simulink model "vx_vy_lifesig_fusion_v2_8a2_long_low_yaw"  (R2024a)
settings: Solver=VariableStepAuto  StartTime=0.0  StopTime=22  RelTol=1e-3
model workspace (MAT data in the model file):
  ax_imu_prereq_Ts = 0.01
  ax_imu_prereq_bias = 0.02
  ax_imu_prereq_fc = 20
  ax_imu_prereq_noise_variance = 2.5e-05
  long_low_yaw_excitation_end_s = 4.5
  long_low_yaw_initial_straight_s = 2
  long_low_yaw_sample_time = 0.01
  long_low_yaw_steer_amplitude_rad = 0.02
  long_low_yaw_steer_frequency_hz = 0.4
  long_low_yaw_steer_profile = [0 0.01 0.02 0.03 0.04 0.05 0.06 0.07 0.08 0.09 0.1 0.11 ... (4402 elements, 2201x2)]
  long_low_yaw_stop_time = 22
  test_steer_amplitude = 0.02
  test_steer_frequency = 0.4
  vy_v17_mode_code = 20
undefined symbols (not defined in the file or in its folder): longitudinal_velocity_estimator_simulink, vy_dynamic_ekf, vy_dynamic_ekf_v1_17_reliability_numeric
libraries: simulink x6, Solver_SF x1
(part 1 of 2)
Description:
  | V2.5 FIXED-WEIGHT INTEGRATION TARGET. Fusion weights [1/3 1/3 1/3] are TEST-ONLY, NOT SELECTED BASELINE WEIGHTS, NOT TUNED, and NOT FROZEN. F P0_F=0.5 and Q_F=0.0025 remain TEST-ONLY, UNTUNED, and UNFROZEN. F feedback_valid_current is fixed false; Vy_FW is observation-only and is not fed back. V2.7 reliability capture role: NON_HOLDOUT_ENGINEERING_DIAGNOSTIC. It is not H01/H02/H03 and must not overwrite formal holdout evidence.
  | V2.7 LIFESIG INTEGRATION TARGET. Independent observation-only LifeSig fusion. Formal fusion inputs are Vy_D/update_valid_D, Vy_K/update_valid_K, Vy_F/propagation_age_steps/age_valid_F, and reset only. NIS, yaw observability, disagreement, covariance, and online truth are excluded. Existing F runtime parameters remain P0_F=0.5 and Q_F=0.0025.
  | V2.8-A2 NON-HOLDOUT LONG-LOW-YAW VALIDATION TARGET. 100-Hz steering: 2.0 s exact zero, one 0.02-rad 0.4-Hz sine period, then 17.5 s exact zero. Vy_true and D/K errors are observation-only diagnostics. No K gate is implemented.
settings Model: Creator=Xiao Hu  LastModifiedBy=21180

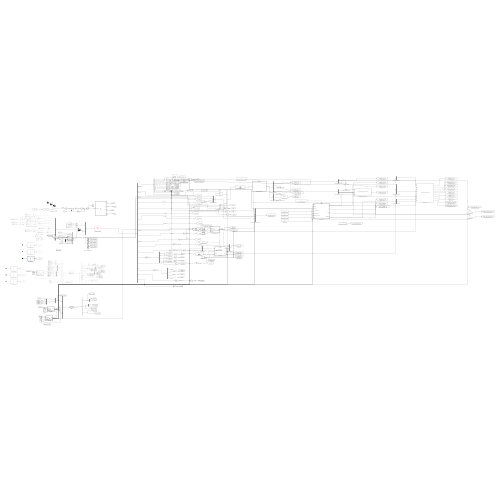
[thumbnail: Simulink's stored preview of the top-level diagram]
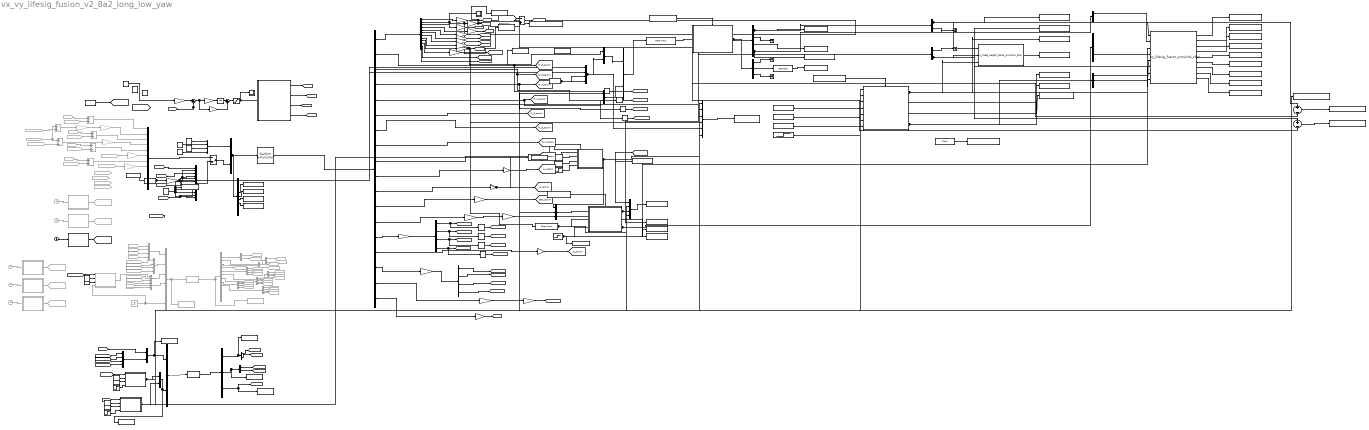
== system vx_vy_lifesig_fusion_v2_8a2_long_low_yaw ==
  note: Product
  AVz传感器 : MATLAB Function  TreatAsAtomicUnit=on  SystemSampleTime=0.01
  Add1 : Sum  Inputs=-+
  Add{4..9} (6 alike) : Sum  Commented=on
  Ax Clean 100Hz Log : ToWorkspace  VariableName=ax_clean_100hz_prereq_log1  SaveFormat=Timeseries  SampleTime=-1
  Ax IMU Bias : Constant  Value=0.02
  Ax IMU Input RT 100Hz : RateTransition  OutPortSampleTime=0.01
  Ax IMU Log : ToWorkspace  VariableName=ax_imu_prereq_log1  SaveFormat=Timeseries  SampleTime=-1
  Ax IMU Reset : Step  Time=0.01  Before=1  After=0  SampleTime=0
  Ax IMU Sensor 100Hz : MATLAB Function  TreatAsAtomicUnit=on  SystemSampleTime=0.01
  Ax IMU White Noise : RandomNumber  Variance=0.000025  Seed=20260820  SampleTime=0.01
  B高附着加速 : MATLAB Function  Commented=on  TreatAsAtomicUnit=on
  CarSim S-Function : Solver_SF/CarSim S-Function  Priority=1  SIMFILE=simfile.sim  Run_RTs=off  vs_state_ind=Run  StopMode_ind=Vehicle Model
  Clock{,1,3..5} (5 alike) : Clock  Commented=on
  Clock2 : Clock
  Constant : Constant  Value=0.02
  Constant1 : Constant  Value=0.02
  Constant{6..10} (5 alike) : Constant  Value=0
  Constant2 : Constant  Value=0.005
  Constant4 : Constant  Value=0.8
  C高附着减速 : MATLAB Function  Commented=on  TreatAsAtomicUnit=on
  D LifeSig Valid Demux : Demux  Outputs=[1 1]
  Demux : Demux  Commented=on  Outputs=[2 2 2 1 4 4 4 4 4 2 2 7]
  Demux{1,9..11,13} (5 alike) : Demux  Commented=on
  Demux12 : Demux  Outputs=[2 2 9]
  Demux14 : Demux  Outputs=2
  Demux18 : Demux  Outputs=2
  Demux2 : Demux  Commented=on  Outputs=2
  Demux3 : Demux
  Demux4 : Demux  Outputs=12
  Demux5 : Demux  Outputs=[12 1 1 1 1 1 1 1 1 1 1 1 1 4 1 4 1 1]
  Demux6 : Demux
  Demux7 : Demux  Commented=on  Outputs=2
  Demux8 : Demux  Commented=on  Outputs=2
  Derivative{,1..4,6..7,12} (8 alike) : Derivative
  D高附着加减速1 : MATLAB Function  TreatAsAtomicUnit=on
  F Feedback Valid Disabled : Constant  Value=0  OutDataTypeStr=double  SampleTime=0.01
  F LifeSig Reliability Demux : Demux  Outputs=[1 1 1]
  F P Feedback Placeholder : Constant  Value=0.5  OutDataTypeStr=double  SampleTime=0.01
  F Reset First Hit : Step  Time=0.01  Before=1  After=0  SampleTime=0.01
  F Vy Feedback Placeholder : Constant  Value=0  OutDataTypeStr=double  SampleTime=0.01
  F-Track 100Hz : Subsystem  TreatAsAtomicUnit=on
  F-Track 100Hz Scheduler : simulink/Ports & Subsystems/Function-Call Generator  sample_time=0.01  numberOfIterations=1  DisallowWideOutput=off
  Fixed Weight D K F Fusion : M-S-Function  FunctionName=vy_fixed_weight_fusion_simulink_sfun  Parameters=0.9004680917645591,1-0.9004680917645591,0
  From : From  Commented=on  GotoTag=weelrate_fl  TagVisibility=global
  From11 : From  Commented=on  GotoTag=weelrate_fr  TagVisibility=global
  From12 : From  Commented=on  GotoTag=W5_T  TagVisibility=global
  From13 : From  Commented=on  GotoTag=W1_T  TagVisibility=global
  From14 : From  Commented=on  GotoTag=weelrate_rl  TagVisibility=global
  From15 : From  Commented=on  GotoTag=weelrate_rr  TagVisibility=global
  From16 : From  Commented=on  GotoTag=WEEL1  TagVisibility=global
  From17 : From  Commented=on  GotoTag=WEEL3  TagVisibility=global
  From18 : From  Commented=on  GotoTag=WEEL2  TagVisibility=global
  From19 : From  Commented=on  GotoTag=WEEL4  TagVisibility=global
  From2 : From  Commented=on  GotoTag=Fd2  TagVisibility=global
  From20 : From  Commented=on  GotoTag=yawrate  TagVisibility=global
  From21 : From  Commented=on  GotoTag=W3_T  TagVisibility=global
  From22 : From  Commented=on  GotoTag=Delta_Torque_rl  TagVisibility=global
  From23 : From  Commented=on  GotoTag=Delta_Torque_fr  TagVisibility=global
  From24 : From  Commented=on  GotoTag=Delta_Torque_rr  TagVisibility=global
  From25 : From  Commented=on  GotoTag=rollrate  TagVisibility=global
  From26 : From  Commented=on  GotoTag=Ay_carsim  TagVisibility=global
  From28 : From  Commented=on  GotoTag=Az_carsim  TagVisibility=global
  From29 : From  Commented=on  GotoTag=W7_T  TagVisibility=global
  From3 : From  Commented=on  GotoTag=Delta_Torque_fl  TagVisibility=global
  From30 : From  Commented=on  GotoTag=pitchrate  TagVisibility=global
  From35 : From  Commented=on  GotoTag=driver_steering
  From39 : From  Commented=on  GotoTag=Delta_Steering_rl  TagVisibility=global
  From4 : From  Commented=on  GotoTag=Fd3  TagVisibility=global
  From42 : From  Commented=on  GotoTag=Delta_Steering_rr  TagVisibility=global
  From43 : From  Commented=on  GotoTag=Fd1  TagVisibility=global
  From5 : From  Commented=on  GotoTag=Delta_Steering_fl  TagVisibility=global
  From50 : From  Commented=on  GotoTag=Fd4  TagVisibility=global
  From6 : From  Commented=on  GotoTag=Delta_Steering_fr  TagVisibility=global
  Fusion D State Select Vy : Demux  Outputs=2
  Fusion D r Terminator : Terminator
  Fusion K State Select Vy : Demux  Outputs=2
  Fusion K Vx Terminator : Terminator
  F低附着加速1 : MATLAB Function  Commented=on  TreatAsAtomicUnit=on
  F低附着加速2 : MATLAB Function  Commented=on  TreatAsAtomicUnit=on
  G0 CarSim Input Demux : Demux  Outputs=16
  G0 Steer Cmd Rad : FromWorkspace  VariableName=long_low_yaw_steer_profile  SampleTime=0.01  Interpolate=off  OutputAfterFinalValue=Holding final value
  Gain{1,10,12,14,17..18,23,29,37} (9 alike) : Gain  Gain=pi/180
  Gain11 : Gain  Gain=1/3.6
  Gain{3,5,9,13} (4 alike) : Gain  Commented=on  Gain=180/pi
  Gain15 : Gain  Gain=1/3.6
  Gain16 : Gain  Gain=9.8
  Gain19 : Gain  Gain=1/16.8
  Gain2 : Gain  Gain=1/16.8
  Gain21 : Gain  Gain=5000
  Gain22 : Gain  Gain=180/pi
  Gain{6..8,24} (4 alike) : Gain  Gain=pi/30
  Gain25 : Gain  Gain=0.07
  Gain28 : Gain  Gain=9.8
  Gain36 : Gain  Gain=9.8
  Gain38 : Gain  Gain=1/3.6
  Gain39 : Gain  Commented=on
  Gain4 : Gain  Gain=1/1000
  Goto10 : Goto  Commented=on  GotoTag=vx_wss  TagVisibility=global
  Goto17 : Goto  Commented=on  GotoTag=P_wss  TagVisibility=global
  Goto28 : Goto  Commented=on  GotoTag=vx_imu  TagVisibility=global
  Goto29 : Goto  Commented=on  GotoTag=P_imu  TagVisibility=global
  Goto30 : Goto  Commented=on  GotoTag=P_wss_imu  TagVisibility=global
  Goto32 : Goto  Commented=on  GotoTag=vx_FL  TagVisibility=global
  Goto38 : Goto  Commented=on  GotoTag=vx_FR  TagVisibility=global
  Goto39 : Goto  Commented=on  GotoTag=vx_RL  TagVisibility=global
  Goto40 : Goto  Commented=on  GotoTag=vx_RR  TagVisibility=global
  Goto41 : Goto  Commented=on  GotoTag=slip_FL  TagVisibility=global
  Goto57 : Goto  Commented=on  GotoTag=slip_FR  TagVisibility=global
  Goto58 : Goto  Commented=on  GotoTag=slip_RL  TagVisibility=global
  Goto59 : Goto  Commented=on  GotoTag=slip_RR  TagVisibility=global
  Goto64 : Goto  Commented=on  GotoTag=rho_FL  TagVisibility=global
  Goto65 : Goto  Commented=on  GotoTag=rho_FR  TagVisibility=global
  Goto66 : Goto  Commented=on  GotoTag=rho_RL  TagVisibility=global
  Goto67 : Goto  Commented=on  GotoTag=rho_RR  TagVisibility=global
  Goto68 : Goto  Commented=on  GotoTag=R_FL  TagVisibility=global
  Goto69 : Goto  Commented=on  GotoTag=R_FR  TagVisibility=global
  Goto7 : Goto  Commented=on  GotoTag=vx_hat  TagVisibility=global
  Goto70 : Goto  Commented=on  GotoTag=R_RL  TagVisibility=global
  Goto71 : Goto  Commented=on  GotoTag=R_RR  TagVisibility=global
  Goto72 : Goto  Commented=on  GotoTag=R_FL  TagVisibility=global
  Goto73 : Goto  Commented=on  GotoTag=R_FR  TagVisibility=global
  Goto74 : Goto  Commented=on  GotoTag=R_RL  TagVisibility=global
  Goto75 : Goto  Commented=on  GotoTag=R_RR  TagVisibility=global
  Goto{76..77,80..82} (5 alike) : Goto  Commented=on  GotoTag=vx_ref  TagVisibility=global
  Goto9 : Goto  Commented=on  GotoTag=P_fused  TagVisibility=global
  G低附着减速2 : MATLAB Function  Commented=on  TreatAsAtomicUnit=on
  H低附着加减速 : MATLAB Function  Commented=on  TreatAsAtomicUnit=on
  Integrator1 : Integrator
  K LifeSig Diagnostic Demux : Demux  Outputs=[1 1 1 1 1 1 1]
  K-KF 100Hz : Subsystem  TreatAsAtomicUnit=on
  K-KF 100Hz Scheduler : simulink/Ports & Subsystems/Function-Call Generator  sample_time=0.01  numberOfIterations=1  DisallowWideOutput=off
  K-KF IMU Mux : Mux  Inputs=3
  K-KF Input Log Mux : Mux
  K-KF P Log : ToWorkspace  VariableName=kkf_P_log1  SaveFormat=Timeseries  SampleTime=-1
  K-KF Reset First Call : Step  Time=0.01  Before=1  After=0  SampleTime=0.01
  K-KF Vx RT 100Hz : RateTransition  OutPortSampleTime=0.01
  K-KF diag Log : ToWorkspace  VariableName=kkf_diag_log1  SaveFormat=Timeseries  SampleTime=-1
  K-KF u Log : ToWorkspace  VariableName=kkf_u_log1  SaveFormat=Timeseries  SampleTime=-1
  K-KF x Log : ToWorkspace  VariableName=kkf_x_log1  SaveFormat=Timeseries  SampleTime=-1
  LifeSig D K F Fusion : M-S-Function  FunctionName=vy_lifesig_fusion_simulink_sfun
  Long Low Yaw D Error : Sum  Inputs=+-
  Long Low Yaw D Error Log : ToWorkspace  VariableName=long_low_yaw_d_error_log  SaveFormat=Timeseries  SampleTime=-1
  Long Low Yaw K Error : Sum  Inputs=+-
  Long Low Yaw K Error Log : ToWorkspace  VariableName=long_low_yaw_k_error_log  SaveFormat=Timeseries  SampleTime=-1
  Long Low Yaw Signed r Log : ToWorkspace  VariableName=long_low_yaw_r_log  SaveFormat=Timeseries  SampleTime=-1
  MATLAB Function5 : MATLAB Function  TreatAsAtomicUnit=on
  Manual Switch1 : ManualSwitch  CurrentSetting=0
  Mux : Mux  Commented=on  Inputs=[4 4 3 3 3 1]
  Mux1 : Mux  Commented=on
  Mux10 : Mux  Inputs=[1 4]
  Mux11 : Mux
  Mux12 : Mux  Inputs=2
  Mux2 : Mux  Commented=on
  Mux3 : Mux  Commented=on  Inputs=3
  Mux4 : Mux  Commented=on  Inputs=3
  Mux5 : Mux  Inputs=12
  Mux6 : Mux
  Mux7 : Mux  Inputs=[4,12]
  Mux8 : Mux  Inputs=12
  Mux9 : Mux  Inputs=[5 2]
  Parallel D Control Mux : Mux  Inputs=[1 4]
  Parallel D Full P Extract : Demux  Outputs=[45 4 22]
  Parallel D Input Mux : Mux  Inputs=[5 2]
  Parallel D Measurement Mux : Mux  Inputs=2
  Parallel D Output Demux : Demux  Outputs=[2 2 65 2]
  Parallel D P 2x2 : Reshape  OutputDimensionality=Customize  OutputDimensions=[2 2]
  Parallel D P Head Terminator : Terminator
  Parallel D P Tail Terminator : Terminator
  Parallel D Pdiag Terminator : Terminator
  Parallel D Rear Steer Zero Rad : Constant  Value=0  OutDataTypeStr=double
  Parallel D Steering Mux : Mux
  Parallel D-EKF 100Hz : Subsystem  TreatAsAtomicUnit=on
  Parallel D-EKF 100Hz Scheduler : simulink/Ports & Subsystems/Function-Call Generator  sample_time=0.01  numberOfIterations=1  DisallowWideOutput=off
  Parallel D-EKF Input RT 100Hz : RateTransition  OutPortSampleTime=0.01
  Parallel Physical Input Log Mux : Mux  Inputs=[1 1 1 1 4 1]
  Random Number : RandomNumber  Variance=0.000025  Seed=20260819  SampleTime=0.01
  Random Number1 : RandomNumber  Variance=0.000025  Seed=20260819  SampleTime=0.01
  Random Number2 : RandomNumber  Variance=0.000025  Seed=20260819  SampleTime=0.01
  Reliability Common Time 100Hz : DigitalClock  SampleTime=0.01
  Reliability Common Time Log : ToWorkspace  VariableName=rel_common_time_100hz_log  SaveFormat=Timeseries  SampleTime=-1
  Reliability D Valid Log : ToWorkspace  VariableName=rel_d_valid_log  SaveFormat=Timeseries  SampleTime=-1
  Reliability F Diagnostic Log : ToWorkspace  VariableName=rel_f_reliability_log  SaveFormat=Timeseries  SampleTime=-1
  Reliability Vy True 100Hz Log : ToWorkspace  VariableName=rel_vy_true_100hz_log  SaveFormat=Timeseries  SampleTime=-1
  Reliability Vy True RT 100Hz : RateTransition  OutPortSampleTime=0.01
  Repeating Sequence Interpolated : simulink/Sources/Repeating Sequence Interpolated  OutValues=[40 40 40 40].'  TimeValues=[0 3 8 16].'  LookUpMeth=Interpolation-Use End Values  tsamp=0.001  OutMin=[]  OutMax=[]  OutDataTypeStr=double  OutputDataTypeScalingMode=double  OutDataType=fixdt(0,8)  OutScaling=2^-10
  Repeating Sequence Interpolated1 : simulink/Sources/Repeating Sequence Interpolated  OutValues=[60 60 60 60].'  TimeValues=[0 3 8 16].'  LookUpMeth=Interpolation-Use End Values  tsamp=0.001  OutMin=[]  OutMax=[]  OutDataTypeStr=double  OutputDataTypeScalingMode=double  OutDataType=fixdt(0,8)  OutScaling=2^-10
  Repeating Sequence Interpolated2 : simulink/Sources/Repeating Sequence Interpolated  OutValues=[72 72 72 72].'  TimeValues=[0 3 8 16].'  LookUpMeth=Interpolation-Use End Values  tsamp=0.001  OutMin=[]  OutMax=[]  OutDataTypeStr=double  OutputDataTypeScalingMode=double  OutDataType=fixdt(0,8)  OutScaling=2^-10
  Saturation : Saturate  UpperLimit=2250  LowerLimit=-2250
  Scope3 : Scope
  Scope8 : Scope
  Step : Step  Commented=on  Time=0.01  Before=1  After=0  SampleTime=0
  Step1 : Step  Time=0.01  Before=1  After=0  SampleTime=0
  Step2 : Step  Time=0.01  Before=1  After=0  SampleTime=0
  Sum3 : Sum  Inputs=|+-
  Sum4 : Sum  Inputs=|++
  To Workspace : ToWorkspace  Commented=on  VariableName=est_y_log  SaveFormat=Timeseries  SampleTime=-1
  To Workspace1 : ToWorkspace  Commented=on  VariableName=est_u_log  SaveFormat=Timeseries  SampleTime=-1
  To Workspace10 : ToWorkspace  VariableName=avz_log1  SaveFormat=Timeseries  SampleTime=-1
  To Workspace2 : ToWorkspace  VariableName=Vx_true_log  SaveFormat=Timeseries  SampleTime=-1
  To Workspace3 : ToWorkspace  VariableName=est_y_log1  SaveFormat=Timeseries  SampleTime=-1
  To Workspace4 : ToWorkspace  VariableName=est_u_log1  SaveFormat=Timeseries  SampleTime=-1
  To Workspace5 : ToWorkspace  VariableName=Vx_true_log2  SaveFormat=Timeseries  SampleTime=-1
  To Workspace6 : ToWorkspace  VariableName=est_z_log1  SaveFormat=Timeseries  SampleTime=-1
  To Workspace7 : ToWorkspace  VariableName=est_diag_log1  SaveFormat=Timeseries  SampleTime=-1
  To Workspace8 : ToWorkspace  VariableName=est_P_log1  SaveFormat=Timeseries  SampleTime=-1
  To Workspace9 : ToWorkspace  VariableName=vy_true_log1  SaveFormat=Timeseries  SampleTime=-1
  avz_imu_g0 : ToWorkspace  VariableName=avz_imu_g0  SaveFormat=Timeseries  SampleTime=-1
      settings: MaxDataPoints=100000
  ay传感器 : MATLAB Function  TreatAsAtomicUnit=on  SystemSampleTime=0.01
  dekf_P_log : ToWorkspace  VariableName=dekf_P_log  SaveFormat=Timeseries  SampleTime=-1
      settings: MaxDataPoints=100000
  dekf_diag_log : ToWorkspace  VariableName=dekf_diag_log  SaveFormat=Timeseries  SampleTime=-1
      settings: MaxDataPoints=100000
  dekf_x_log : ToWorkspace  VariableName=dekf_x_log  SaveFormat=Timeseries  SampleTime=-1
      settings: MaxDataPoints=100000
  fusion_f_P_log : ToWorkspace  VariableName=fusion_f_P_log  SaveFormat=Timeseries  SampleTime=-1
  fusion_f_diag_log : ToWorkspace  VariableName=fusion_f_diag_log  SaveFormat=Timeseries  SampleTime=-1
  fusion_vy_d_log : ToWorkspace  VariableName=fusion_vy_d_log  SaveFormat=Timeseries  SampleTime=-1
  fusion_vy_f_log : ToWorkspace  VariableName=fusion_vy_f_log  SaveFormat=Timeseries  SampleTime=-1
  fusion_vy_fw_log : ToWorkspace  VariableName=fusion_vy_fw_log  SaveFormat=Timeseries  SampleTime=-1
  fusion_vy_k_log : ToWorkspace  VariableName=fusion_vy_k_log  SaveFormat=Timeseries  SampleTime=-1
  lifesig_alpha_d_log : ToWorkspace  VariableName=lifesig_alpha_d_log  SaveFormat=Timeseries  SampleTime=-1
  lifesig_alpha_f_log : ToWorkspace  VariableName=lifesig_alpha_f_log  SaveFormat=Timeseries  SampleTime=-1
  lifesig_alpha_k_log : ToWorkspace  VariableName=lifesig_alpha_k_log  SaveFormat=Timeseries  SampleTime=-1
  lifesig_fallback_active_log : ToWorkspace  VariableName=lifesig_fallback_active_log  SaveFormat=Timeseries  SampleTime=-1
  lifesig_fusion_valid_log : ToWorkspace  VariableName=lifesig_fusion_valid_log  SaveFormat=Timeseries  SampleTime=-1
  lifesig_h_d_log : ToWorkspace  VariableName=lifesig_h_d_log  SaveFormat=Timeseries  SampleTime=-1
  lifesig_h_f_log : ToWorkspace  VariableName=lifesig_h_f_log  SaveFormat=Timeseries  SampleTime=-1
  lifesig_h_k_log : ToWorkspace  VariableName=lifesig_h_k_log  SaveFormat=Timeseries  SampleTime=-1
  lifesig_vy_ls_log : ToWorkspace  VariableName=lifesig_vy_ls_log  SaveFormat=Timeseries  SampleTime=-1
  parallel_input_log : ToWorkspace  VariableName=parallel_input_log  SaveFormat=Timeseries  SampleTime=-1
      settings: MaxDataPoints=100000
  reset_g0 : ToWorkspace  VariableName=reset_g0  SaveFormat=Timeseries  SampleTime=-1
      settings: MaxDataPoints=100000
  steer_cmd_rad : ToWorkspace  VariableName=steer_cmd_rad  SaveFormat=Timeseries  SampleTime=-1
      settings: MaxDataPoints=100000
  steer_fl_carsim_deg : ToWorkspace  VariableName=steer_fl_carsim_deg  SaveFormat=Timeseries  SampleTime=-1
      settings: MaxDataPoints=100000
  steer_fr_carsim_deg : ToWorkspace  VariableName=steer_fr_carsim_deg  SaveFormat=Timeseries  SampleTime=-1
      settings: MaxDataPoints=100000
  steer_rl_carsim_deg : ToWorkspace  VariableName=steer_rl_carsim_deg  SaveFormat=Timeseries  SampleTime=-1
      settings: MaxDataPoints=100000
  steer_rr_carsim_deg : ToWorkspace  VariableName=steer_rr_carsim_deg  SaveFormat=Timeseries  SampleTime=-1
      settings: MaxDataPoints=100000
  steer_to_carsim_deg : ToWorkspace  VariableName=steer_to_carsim_deg  SaveFormat=Timeseries  SampleTime=-1
      settings: MaxDataPoints=100000
  估计vx : MATLABFcn  Commented=on  MATLABFcn=longitudinal_velocity_estimator_simulink(u)  OutputDimensions=38
  估计vy : MATLABFcn  MATLABFcn=vy_dynamic_ekf(u)  OutputDimensions=13
  tag scope: Ax_carsim=global, Ay_carsim=global, Az_carsim=global, Fx_fl_carsim=global, Fx_fr_carsim=global, Fx_rl_carsim=global, Fx_rr_carsim=global, Fy_fl_carsim=global, Fy_fr_carsim=global, Fy_rl_carsim=global, Fy_rr_carsim=global, P_r=global, P_vy=global, Vx=global, Vy=global, Vy_hat=global, W1_T=global, W3_T=global, W5_T=global, W7_T=global, WEEL1=global, WEEL2=global, WEEL3=global, WEEL4=global, beta_carsim=global, delta_zs1=global, delta_zs2=global, delta_zs3=global, delta_zs4=global, delta_zsd1=global, delta_zsd2=global, delta_zsd3=global, delta_zsd4=global, diag_out=global, driver_steering10=global, driver_steering5=global, e_yawrate=global, fyd1=global, fyd2=global, fyd3=global, fyd4=global, mu=global, pitchrate=global, r_hat=global, roll=global, rollrate=global, vx_ref=global, weelrate_fl=global, weelrate_fr=global, weelrate_rl=global, weelrate_rr=global, x_carsim=global, y_carsim=global, yaw_carsim=global, yawrate=global
  wires:
  From13/1 -> Add4/1
  Gain14/1 -> Gain2/1  "beta_carsim"
  Add1/1 -> [e_yawrate]  "e_yawrate"
  Gain3/1 -> Mux5/4
  From6/1 -> Add8/2  "delta3"
  [W1_T] -> Mux8/1
  Demux5/7 -> [Fx_fr_carsim]  "Fzfr_carsim"
  Demux3/4 -> Derivative3/1, [delta_zs4]
  From12/1 -> Add6/1
  From35/1 -> Add9/1, Add8/1
  Gain39/1 -> Gain5/1
  Gain13/1 -> Mux5/8
  Demux6/4 -> [WEEL4]  "WEEL4"
  Constant6/1 -> Mux6/2
  Add9/1 -> Gain39/1  "总的转角1"
  Derivative1/1 -> [delta_zsd2]
  Demux5/12 -> Gain29/1
  Demux5/8 -> [Fx_rl_carsim]  "Fzrl_carsim"
  Gain19/1 -> [driver_steering10]  "ds1"
  Add4/1 -> Mux5/1  "T1"
  Gain4/1 -> Demux3/1
  Gain38/1 -> To Workspace2/1, [Vx], K-KF Vx RT 100Hz/1, Parallel D Control Mux/1, Parallel Physical Input Log Mux/4, F-Track 100Hz/3(Vx_source)  "vx_carsim"
  Gain8/1 -> [weelrate_rr]  "weelrate4"
  Add5/1 -> Mux5/3  "T2"
  Demux6/3 -> [WEEL2]  "WEEL2"
  Mux7/1 -> CarSim S-Function/1, G0 CarSim Input Demux/1  "u"
  Mux8/1 -> Manual Switch1/2  "u"
  From21/1 -> Add5/1
  MATLAB Function5/2(Tor_R1) -> [W3_T]  "T_R1"
  Gain36/1 -> [Ay_carsim]  "Ay_carsim"
  Derivative3/1 -> [delta_zsd4]
  Gain11/1 -> To Workspace9/1, [Vy], Reliability Vy True RT 100Hz/1  "Vy"
  Sum4/1 -> Saturation/1
  Gain9/1 -> Mux5/6
  Demux5/4 -> Derivative6/1, [Fy_rl_carsim]  "Fyrl_carsim"
  Gain5/1 -> Mux5/2
  Demux5/16 -> Gain17/1
  Gain21/1 -> Sum4/2
  CarSim S-Function/1 -> Demux5/1
  Derivative4/1 -> [fyd2]
  From39/1 -> Gain9/1
  From22/1 -> Add6/2  "delta3"
  Derivative12/1 -> [fyd1]
  From23/1 -> Add5/2  "delta2"
  Gain18/1 -> Gain19/1  "beta_carsim"
  Gain7/1 -> [weelrate_rl]  "weelrate3"
  Derivative7/1 -> [fyd4]
  Derivative6/1 -> [fyd3]
  Constant9/1 -> Mux6/3
  Mux6/1 -> Mux7/1  "u"
  [W3_T] -> Mux8/3  "q1"
  Gain12/1 -> [roll]  "roll"
  Gain17/1 -> Demux6/1
  Demux5/17 -> Gain18/1
  Demux6/2 -> [WEEL3]  "WEEL3"
  Gain16/1 -> [Az_carsim]  "Ax_carsim"
  Derivative/1 -> [delta_zsd1]
  Demux6/1 -> [WEEL1]  "WEEL1"
  Constant10/1 -> Mux8/12, Mux8/11, Mux8/10, Mux8/6, Mux8/8, Mux8/9
  MATLAB Function5/4(Tor_R2) -> [W7_T]  "T_R2"
  Demux5/13 -> Gain14/1
  Add6/1 -> Mux5/5  "T3"
  From5/1 -> Add9/2
  From3/1 -> Add4/2  "delta1"
  Demux4/7 -> Gain7/1
  MATLAB Function5/1(Tor_L1) -> [W1_T]  "T_L1"
  Demux3/3 -> Derivative2/1, [delta_zs3]
  Demux5/6 -> [Fx_fl_carsim]  "Fzfl_carsim"
  Constant4/1 -> [mu]
  Integrator1/1 -> Sum4/1
  Demux4/3 -> Gain12/1
  Demux5/5 -> [Fy_rr_carsim], Derivative7/1  "Fyrr_carsim"
  Demux4/6 -> Gain6/1
  Derivative2/1 -> [delta_zsd3]
  Gain2/1 -> [driver_steering5]  "ds"
  Demux4/11 -> [x_carsim]  "X"
  Constant8/1 -> Mux6/4
  Demux5/2 -> Derivative12/1, [Fy_fl_carsim]  "Fyfl_carsim"
  Gain6/1 -> [weelrate_fr]  "weelrate2"
  Demux5/1 -> Demux4/1  "delta_carsim"
  Demux5/11 -> Gain28/1  "w_rl_carsim"
  Demux4/5 -> Gain24/1
  Demux5/14 -> Gain4/1
  Add7/1 -> Mux5/7  "T4"
  Manual Switch1/1 -> Mux7/2  "add_Mz"
  Demux5/3 -> Derivative4/1, [Fy_fr_carsim]  "Fyfr_carsim"
  From24/1 -> Add7/2
  Demux4/12 -> [y_carsim]  "Y"
  Demux4/4 -> Gain23/1
  Demux4/2 -> Scope3/1, To Workspace10/1, Gain10/1
  Demux4/8 -> Gain8/1
  Demux5/10 -> Gain36/1  "Ay_carsim"
  Gain25/1 -> Integrator1/1
  Demux3/2 -> Derivative1/1, [delta_zs2]
  From29/1 -> Add7/1  "delta4"
  Gain37/1 -> [yaw_carsim]  "yaw_carsim"
  [driver_steering] -> ?
  Demux4/9 -> Gain38/1
  Demux3/1 -> Derivative/1, [delta_zs1]
  [W7_T] -> Mux8/7  "q1"
  [Vx] -> Sum3/2  "vx"
  Demux5/15 -> Gain16/1  "w_rl_carsim"
  Demux4/1 -> Gain11/1
  Gain28/1 -> [Ax_carsim], Ax IMU Input RT 100Hz/1  "Ax_carsim"
  Gain24/1 -> [weelrate_fl]  "轮速实际值"
  From42/1 -> Gain13/1
  Constant7/1 -> Mux6/1
  Gain22/1 -> Mux8/2, Mux8/4, steer_to_carsim_deg/1
  Gain10/1 -> Add1/2, [yawrate]  "yawrate"
  [W5_T] -> Mux8/5
  Gain29/1 -> [beta_carsim]  "beta_carsim"
  Sum3/1 -> Gain25/1, Gain21/1
  Gain23/1 -> [rollrate]  "rollrate"
  MATLAB Function5/3(Tor_L2) -> [W5_T]  "T_L2"
  Mux5/1 -> Manual Switch1/1  "u"
  Add8/1 -> Gain3/1  "总的转角2"
  Demux4/10 -> Gain37/1
  Demux5/9 -> [Fx_rr_carsim]  "Fzrr_carsim"
  [yawrate_ref] -> Add1/1
  Mux/1 -> 估计vx/1, To Workspace1/1
  Mux1/1 -> Mux/1
  From/1 -> Mux1/1
  From11/1 -> Mux1/2
  From14/1 -> Mux1/3
  From15/1 -> Mux1/4
  From16/1 -> Mux2/1
  From17/1 -> Mux2/2
  From18/1 -> Mux2/3
  From19/1 -> Mux2/4
  Mux2/1 -> Mux/2
  Mux3/1 -> Mux/3
  Mux4/1 -> Mux/4
  Gain1/1 -> [pitchrate]  "pitchrate"
  Demux5/18 -> Gain1/1
  [Ax_carsim] -> F低附着加速2/1(axCarsim)
  From26/1 -> Mux3/2
  From28/1 -> Mux3/3
  From20/1 -> Mux4/1
  From30/1 -> Mux4/2
  From25/1 -> Mux4/3
  估计vx/1 -> Demux/1, To Workspace/1  "T_L1"
  Demux/1 -> Demux2/1
  Demux2/1 -> Goto7/1
  Demux2/2 -> Goto9/1
  Demux7/1 -> Goto10/1
  Demux/2 -> Demux7/1
  Demux7/2 -> Goto17/1
  Demux/3 -> Demux8/1
  Demux8/2 -> Goto29/1
  Demux8/1 -> Goto28/1
  Demux/4 -> Goto30/1
  Demux1/1 -> Goto32/1
  Demux1/2 -> Goto38/1
  Demux1/3 -> Goto39/1
  Demux1/4 -> Goto40/1
  Demux/5 -> Demux1/1
  Demux9/3 -> Goto58/1
  Demux/6 -> Demux9/1
  Demux9/4 -> Goto59/1
  Demux9/2 -> Goto57/1
  Demux9/1 -> Goto41/1
  Demux/7 -> Demux10/1
  Demux10/3 -> Goto66/1
  Demux10/1 -> Goto64/1
  Demux10/4 -> Goto67/1
  Demux10/2 -> Goto65/1
  Demux11/3 -> Goto70/1
  Demux11/4 -> Goto71/1
  Demux/8 -> Demux11/1
  Demux11/2 -> Goto69/1
  Demux11/1 -> Goto68/1
  Demux13/2 -> Goto73/1
  Demux/9 -> Demux13/1
  Demux13/3 -> Goto74/1
  Demux13/4 -> Goto75/1
  Demux13/1 -> Goto72/1
  Step/1 -> F低附着加速2/4(resetFlag), Mux/6
  Repeating Sequence Interpolated2/1 -> Gain15/1  "theta_des"
  Gain15/1 -> Sum3/1  "Vy"
  Clock/1 -> B高附着加速/1(t)
  B高附着加速/1(vref) -> Goto76/1  "T_L1"
  C高附着减速/1(Vx_ref) -> Goto77/1  "T_L1"
  Clock1/1 -> C高附着减速/1(t)
  Clock2/1 -> D高附着加减速1/1(t)
  D高附着加减速1/1(Vx_ref) -> [vx_ref]  "T_L1"
  Clock3/1 -> F低附着加速1/1(t)
  F低附着加速1/1(vref) -> Goto80/1  "T_L1"
  Saturation/1 -> Scope8/1, MATLAB Function5/1(Drive_torque)
  G低附着减速2/1(vref) -> Goto81/1  "T_L1"
  Clock4/1 -> G低附着减速2/1(t)
  H低附着加减速/1(vref) -> Goto82/1  "T_L1"
  Clock5/1 -> H低附着加减速/1(t)
  Constant/1 -> F低附着加速2/3(biasInput)
  Random Number/1 -> F低附着加速2/2(whiteNoise)
  F低附着加速2/1(axOut) -> Mux3/1  "T_L1"
  [Ay_carsim] -> ay传感器/1(ayCarsim)
  估计vy/1 -> Demux12/1  "T_L1"
  Demux18/2 -> [r_hat]
  Demux12/3 -> [diag_out], To Workspace7/1
  Demux12/1 -> To Workspace3/1, Demux18/1
  Step1/1 -> ay传感器/4(resetFlag)
  Constant1/1 -> ay传感器/3(biasInput)
  [WEEL3] -> Mux11/3
  [WEEL4] -> Mux11/4
  Random Number1/1 -> ay传感器/2(whiteNoise)
  [WEEL2] -> Mux11/2
  Mux9/1 -> 估计vy/1
  [WEEL1] -> Mux11/1
  Mux11/1 -> Mux10/2
  [Vx] -> Mux10/1
  Mux10/1 -> To Workspace4/1, Mux9/1
  ay传感器/1(ayOut) -> Mux12/1, K-KF IMU Mux/2, K-KF Input Log Mux/2, Parallel D Measurement Mux/1, Parallel Physical Input Log Mux/2, F-Track 100Hz/1(Ay_IMU)  "Ay_IMU"
  Mux12/1 -> Mux9/2, To Workspace6/1
  Random Number2/1 -> AVz传感器/2(whiteNoise)
  Constant2/1 -> AVz传感器/3(biasInput)
  Step2/1 -> AVz传感器/4(resetFlag)
  [yawrate] -> AVz传感器/1(rCarsim)
  AVz传感器/1(rOut) -> Mux12/2, K-KF IMU Mux/3, K-KF Input Log Mux/3, avz_imu_g0/1, Parallel D Measurement Mux/2, Parallel Physical Input Log Mux/3, F-Track 100Hz/2(AVz_IMU), Long Low Yaw Signed r Log/1  "AVz_IMU"
  Demux18/1 -> [Vy_hat]
  Demux14/2 -> [P_r]
  Demux14/1 -> [P_vy]
  Demux12/2 -> To Workspace8/1, Demux14/1
  Ax IMU Input RT 100Hz/1 -> Ax IMU Sensor 100Hz/1(axCarsim), Ax Clean 100Hz Log/1
  Ax IMU White Noise/1 -> Ax IMU Sensor 100Hz/2(whiteNoise)
  Ax IMU Bias/1 -> Ax IMU Sensor 100Hz/3(biasInput)
  Ax IMU Reset/1 -> Ax IMU Sensor 100Hz/4(resetFlag)
  Ax IMU Sensor 100Hz/1(axOut) -> [Ax_IMU], Ax IMU Log/1, K-KF IMU Mux/1, K-KF Input Log Mux/1, Parallel Physical Input Log Mux/1  "Ax_IMU"
  K-KF IMU Mux/1 -> K-KF 100Hz/1(u)
  K-KF Vx RT 100Hz/1 -> K-KF 100Hz/2(Vx_meas), K-KF Input Log Mux/4
  K-KF Reset First Call/1 -> K-KF 100Hz/3(resetFlag), reset_g0/1, Parallel Physical Input Log Mux/6, LifeSig D K F Fusion/8
  K-KF 100Hz Scheduler/1 -> K-KF 100Hz/Trigger
  K-KF Input Log Mux/1 -> K-KF u Log/1
  K-KF 100Hz/1(x_hat) -> K-KF x Log/1, Fusion K State Select Vy/1
  K-KF 100Hz/2(P) -> K-KF P Log/1
  K-KF 100Hz/3(diag_out) -> K-KF diag Log/1, K LifeSig Diagnostic Demux/1
  G0 CarSim Input Demux/6 -> steer_fl_carsim_deg/1
  G0 CarSim Input Demux/8 -> steer_fr_carsim_deg/1
  G0 CarSim Input Demux/10 -> steer_rl_carsim_deg/1
  G0 CarSim Input Demux/12 -> steer_rr_carsim_deg/1
  Parallel D Rear Steer Zero Rad/1 -> Parallel D Steering Mux/3, Parallel D Steering Mux/4
  Parallel D Steering Mux/1 -> Parallel D Control Mux/2, Parallel Physical Input Log Mux/5
  Parallel D Control Mux/1 -> Parallel D Input Mux/1
  Parallel D Measurement Mux/1 -> Parallel D Input Mux/2
  Parallel D Input Mux/1 -> Parallel D-EKF Input RT 100Hz/1
  Parallel D-EKF Input RT 100Hz/1 -> Parallel D-EKF 100Hz/1(In1)
  Parallel D-EKF 100Hz Scheduler/1 -> Parallel D-EKF 100Hz/Trigger
  Parallel D-EKF 100Hz/1(Out1) -> Parallel D Output Demux/1, Parallel D Full P Extract/1
  Parallel D Output Demux/2 -> Parallel D Pdiag Terminator/1
  Parallel D Full P Extract/1 -> Parallel D P Head Terminator/1
  Parallel D Full P Extract/2 -> Parallel D P 2x2/1
  Parallel D Full P Extract/3 -> Parallel D P Tail Terminator/1
  Parallel D Output Demux/1 -> dekf_x_log/1, Fusion D State Select Vy/1
  Parallel D P 2x2/1 -> dekf_P_log/1
  Parallel D Output Demux/3 -> dekf_diag_log/1
  Parallel Physical Input Log Mux/1 -> parallel_input_log/1
  F-Track 100Hz Scheduler/1 -> F-Track 100Hz/Trigger
  F Vy Feedback Placeholder/1 -> F-Track 100Hz/4(Vy_feedback_current)
  F P Feedback Placeholder/1 -> F-Track 100Hz/5(P_feedback_current)
  F Feedback Valid Disabled/1 -> F-Track 100Hz/6(feedback_valid_current)
  F Reset First Hit/1 -> F-Track 100Hz/7(reset)
  Fusion D State Select Vy/1 -> Fixed Weight D K F Fusion/1, fusion_vy_d_log/1, LifeSig D K F Fusion/1, Long Low Yaw D Error/1
  Fusion K State Select Vy/2 -> Fixed Weight D K F Fusion/2, fusion_vy_k_log/1, LifeSig D K F Fusion/3, Long Low Yaw K Error/1
  F-Track 100Hz/1(Vy_F) -> Fixed Weight D K F Fusion/3, fusion_vy_f_log/1, LifeSig D K F Fusion/5
  F-Track 100Hz/2(P_F) -> fusion_f_P_log/1
  F-Track 100Hz/3(diag_F) -> fusion_f_diag_log/1
  Fixed Weight D K F Fusion/1 -> fusion_vy_fw_log/1
  Fusion D State Select Vy/2 -> Fusion D r Terminator/1
  Fusion K State Select Vy/1 -> Fusion K Vx Terminator/1
  Parallel D Output Demux/4 -> Reliability D Valid Log/1, D LifeSig Valid Demux/1
  F-Track 100Hz/4(ReliabilityDiag) -> Reliability F Diagnostic Log/1, F LifeSig Reliability Demux/1
  Reliability Vy True RT 100Hz/1 -> Reliability Vy True 100Hz Log/1, Long Low Yaw D Error/2, Long Low Yaw K Error/2
  Reliability Common Time 100Hz/1 -> Reliability Common Time Log/1
  D LifeSig Valid Demux/1 -> LifeSig D K F Fusion/2
  K LifeSig Diagnostic Demux/6 -> LifeSig D K F Fusion/4
  F LifeSig Reliability Demux/1 -> LifeSig D K F Fusion/6
  F LifeSig Reliability Demux/2 -> LifeSig D K F Fusion/7
  LifeSig D K F Fusion/1 -> lifesig_vy_ls_log/1
  LifeSig D K F Fusion/2 -> lifesig_alpha_d_log/1
  LifeSig D K F Fusion/3 -> lifesig_alpha_k_log/1
  LifeSig D K F Fusion/4 -> lifesig_alpha_f_log/1
  LifeSig D K F Fusion/5 -> lifesig_h_d_log/1
  LifeSig D K F Fusion/6 -> lifesig_h_k_log/1
  LifeSig D K F Fusion/7 -> lifesig_h_f_log/1
  LifeSig D K F Fusion/8 -> lifesig_fusion_valid_log/1
  LifeSig D K F Fusion/9 -> lifesig_fallback_active_log/1
  G0 Steer Cmd Rad/1 -> Gain22/1, steer_cmd_rad/1, Parallel D Steering Mux/1, Parallel D Steering Mux/2
  Long Low Yaw D Error/1 -> Long Low Yaw D Error Log/1
  Long Low Yaw K Error/1 -> Long Low Yaw K Error Log/1
